simulink model "Lab02"  (Simulink 6.3)
settings: Solver=ode45  StartTime=0.0  StopTime=10.0  RelTol=1e-3
libraries: simulink x1
settings Model: LastModifiedBy=Frank Gloria

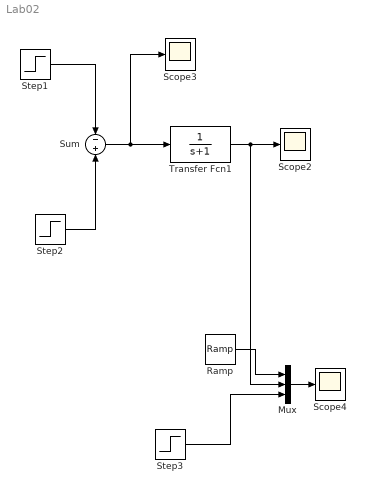
== system Lab02 ==
  Mux : Mux  Inputs=3
  Ramp : simulink/Sources/Ramp  slope=1  start=0  X0=0
  Scope2 : Scope
      settings: SaveName=ScopeData2
  Scope3 : Scope
      settings: SaveName=ScopeData3
  Scope4 : Scope
      settings: SaveName=ScopeData4
  Step1 : Step  Time=0.2  After=0  SampleTime=0
  Step2 : Step  Time=0  SampleTime=0
  Step3 : Step  Time=0  SampleTime=0
  Sum : Sum  Inputs=-+
  Transfer Fcn1 : TransferFcn  Numerator=1  Denominator=[1 1]
  wires:
  Step2/1 -> Sum/2
  Sum/1 -> Transfer Fcn1/1, Scope3/1
  Transfer Fcn1/1 -> Scope2/1, Mux/2
  Step1/1 -> Sum/1
  Ramp/1 -> Mux/1
  Step3/1 -> Mux/3
  Mux/1 -> Scope4/1
